simulink model "SG__MDL_IO104_IO135"  (R2022b)
settings: Solver=FixedStepAuto  StartTime=0.0  StopTime=Inf  RelTol=1e-3  EnableMultiTasking=on
model workspace (MAT data in the model file):
  a = 0.28
  ff = 1200
  fi = 150
  tmax = 40
undefined symbols (not defined in the file or in its folder): Ended, Single
libraries: dspsigops x11, simulink x8, speedgoatlib_IO135 x3, speedgoatlib_IO104 x3, hdlsllib x2, slrealtimeloglib x1, dspsrcs4 x1
settings Model: SimulationMode=external  Creator=padlewsk  LastModifiedBy=padlewsk
settings SolverCC: ConcurrentTasks=on  AlgebraicLoopSolver=TrustRegion  PositivePriorityOrder=on  AutoInsertRateTranBlk=on
settings DataIOCC: SaveFormat=StructureWithTime
settings OptimizationCC: BlockReduction=off  OptimizeBlockIOStorage=off
settings DebuggingCC: TasksWithSamePriorityMsg=none  UnconnectedInputMsg=warning  UnconnectedOutputMsg=warning  UnconnectedLineMsg=warning
settings HardwareCC: ProdBitPerLong=64  ProdLongLongMode=on  ProdHWDeviceType=Intel->x86-64 (Linux 64)
settings ModelReferenceCC: EnableRefExpFcnMdlSchedulingChecks=on
settings RTWCC: Description=Simulink Real-Time  SystemTargetFile=slrealtime.tlc  TemplateMakefile=slrealtime_default_tmf  Toolchain=Simulink Real-Time Toolchain  BuildConfiguration=Faster Runs  CodeExecutionProfiling=on  TargetLang=C++

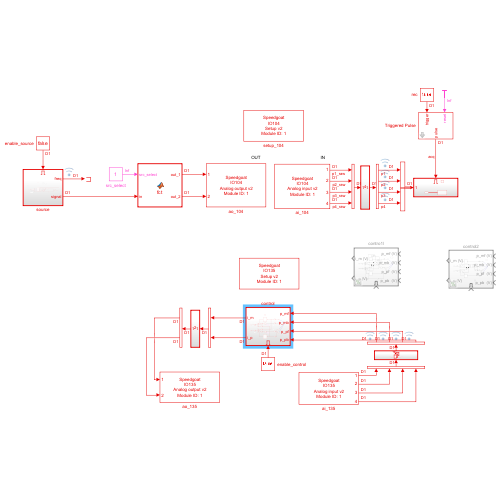
[thumbnail: Simulink's stored preview of the top-level diagram]
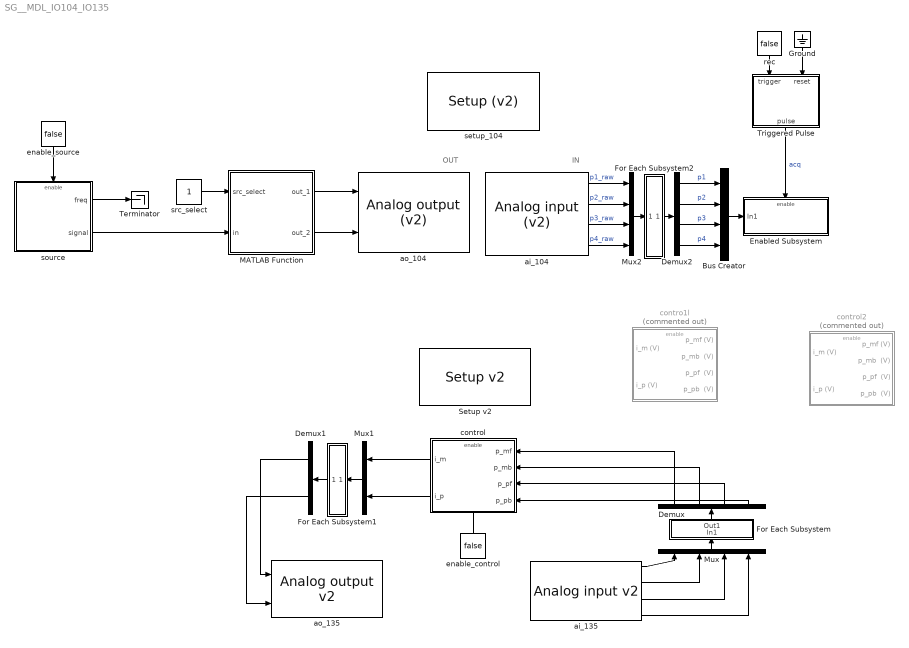
== system SG__MDL_IO104_IO135 ==
  note: IN
  note: OUT
  Bus Creator : BusCreator  Inputs=4
  Demux : Demux
  Demux1 : Demux  Outputs=2
  Demux2 : Demux
  Enabled Subsystem : Subsystem  TreatAsAtomicUnit=on
  For Each Subsystem : Subsystem  TreatAsAtomicUnit=on
  For Each Subsystem1 : Subsystem  TreatAsAtomicUnit=on
  For Each Subsystem2 : Subsystem  TreatAsAtomicUnit=on
  Ground : Ground
  MATLAB Function : MATLAB Function  TreatAsAtomicUnit=on
  Mux : Mux
  Mux1 : Mux  Inputs=2
  Mux2 : Mux
  "Setup v2 " : speedgoatlib_IO135/Setup v2   parPciSlot=-1  parModuleId=1  parInterModuleSync=None  parConvClockBaseRate=20MHz  parConvClock1Divider=20000  parConvClock2Divider=20000  parFrameTriggerEnable=off  parFrameTriggerDivider=10  parConvClock1BaseRate=1  parConvClock2BaseRate=1  parFrameTriggerClock=1  parAdcChannels=[1:4]  parAdcRange1=+-5V  parAdcRange2=+-5V  parAdcRange3=+-5V  parAdcRange4=+-5V  parAdcVoltageRange=[1 1 1 1]  parAdcOversampling1=None  parAdcOversampling2=None  parAdcOversampling3=None  parAdcOversampling4=None  parAdcOversamplRate=[1 1 1 1]  parAdcAutoCorrection=on  parAdcContSampling=off  parAdcDmaEnable=off  parAdcDmaClock=Clock 1  parAdcFrameSize_=100  parAdcSampleTime_=-1  parAdcActiveDmaDevices=[1 1 1 1]  parAdcFrameTriggerEnable=0  parAdcFrameSize=100  parAdcSampleTime=0.1  parDacChannels=[1 2]  parDacInitValues=0  parDacReset=1  parDacRange1=+-10V  parDacRange2=+-10V  parDacRange3=+-10V  parDacRange4=+-10V  parDacRange5=+-10V  parDacRange6=+-10V  parDacRange7=+-10V  parDacRange8=+-10V  parDacRange9=+-10V  parDacRange10=+-10V  parDacRange11=+-10V  parDacRange12=+-10V  parDacRange13=+-10V  parDacRange14=+-10V  parDacRange15=+-10V  parDacRange16=+-10V  parDacVoltageRange=[5 5 5 5 5 5 5 5 5 5 5 5 5 5 5 5]  parDacAutoCorrection=on  parDacSyncOut=on  parDacDmaEnable=off  parDacDmaLatency=Until next frame  parDacDmaClock=Clock 1  parDacFrameSize_=100  parDacSampleTime_=-1  parDacActiveDmaDevices=[1 1 1 1]  parDacFrameTriggerEnable=0  parDacFrameSize=100  parDacSampleTime=0.1  parDoChannels=[]  parDoInitValues=0  parDoReset=1  parDiChannels=[]  parDiDebounceEnable=off  parDiDebounceTime=0  parDiDebounceValue=0  parDioPullRefFront=Pull-up 3.3V  parDioPullRefRear=Floating
      settings: SourceProductName=Simulink Real-Time: Speedgoat I/O Blockset
  Terminator : Terminator
  Triggered Pulse : Subsystem  mask(Triggered Pulse){N=4}
      mask prompts: N "Length (N samples)"
      mask help: Generates a single pulse of N samples length
  ai_104 : speedgoatlib_IO104/Analog input (v2)   parModuleId=1  parTs=5e-05  parPciSlot=-1  parAdChannels=[1,2,3,4]  parAdChannelsSorted=[1,2,3,4]  parAdRange1=+-2.5V  parAdRange2=+-2.5V  parAdCoupling=Single-Ended  parAdFrameSize=1  parAdUseTrigger=off  parAdClockInitiator=Initiator  parAdSampleTime=9.920634921e-07  parTriggerInitiator=Initiator  parTriggerRate=4.161015625e-01
      settings: SourceProductName=Simulink Real-Time: Speedgoat I/O Blockset
  ai_135 : speedgoatlib_IO135/Analog input v2   parModuleId=1  parSampleTime=5e-05  parPciSlot=-1  parAdcChannels=[1 2 3 4]  parAdcVoltageRange=[1 1 1 1]  parAdcOversamplRate=[1 1 1 1]  parAdcContSampling=0  parAdcDmaEnable=0  parAdcActiveDmaDevices=[1 1 1 1]  parAdcFrameSize=100
      settings: SourceProductName=Simulink Real-Time: Speedgoat I/O Blockset
  ao_104 : speedgoatlib_IO104/Analog output (v2)   parModuleId=1  parTs=5e-05  parPciSlot=-1  parDaChannels=[1,2]  parDaChannelsSorted=[1,2]  parDaInitValue=[0,0]  parDaReset=[1,1]  parDaRange=+-10V  parDaFrameSize=1  parDaUseTrigger=off  parDaClockInitiator=Initiator  parDaSampleTime=9.920634921e-07  parTriggerInitiator=Initiator  parTriggerRate=4.161015625e-01  parAdBlockPresent=1
      settings: SourceProductName=Simulink Real-Time: Speedgoat I/O Blockset
  ao_135 : speedgoatlib_IO135/Analog output v2   parModuleId=1  parSampleTime=5e-05  parPciSlot=-1  parDacChannels=[1 2]  parDacVoltageRange=[5 5 5 5 5 5 5 5 5 5 5 5 5 5 5 5]  parDacInitValues=[0 0]  parDacReset=[1 1]  parDacSyncOut=1  parDacDmaEnable=0  parDacActiveDmaDevices=[1 1 1 1]  parDacDmaLatency=2  parDacFrameSize=100
      settings: SourceProductName=Simulink Real-Time: Speedgoat I/O Blockset
  contro1l : Subsystem  Commented=on
  control : Subsystem
  control2 : Subsystem  Commented=on
  enable_control : Constant  Value=false  SampleTime=-1
  enable_source : Constant  Value=false  SampleTime=-1
  rec : Constant  Value=false  SampleTime=-1
  setup_104 : speedgoatlib_IO104/Setup (v2)   parPciSlot=-1  parModuleId=1  parTriggerInitiator=Initiator  parTriggerRate=4.161015625e-01  parCalibrate=off  parAdChannels=[1:4]  parAdRange1=+-2.5V  parAdRange2=+-2.5V  parAdCoupling=Single-Ended  parAdUseTrigger=off  parAdFrameSize=1  parAdClockInitiator=Initiator  parAdSampleTime=9.920634921e-07  parDaChannels=[1:2]  parDaChannelsSorted=[1,2]  parDaInitValue=[0]  parDaReset=[1]  parDaRange=+-10V  parDaUseTrigger=off  parDaFrameSize=1  parDaClockInitiator=Initiator  parDaSampleTime=9.920634921e-07  parDioByte0Dir=Outputs  parDioByte1Dir=Inputs  parDoChannels=[]  parDoInitValues=[0]  parDoReset=[1]  parDiChannels=[]
      settings: SourceProductName=Simulink Real-Time: Speedgoat I/O Blockset
  source : Subsystem  TreatAsAtomicUnit=on
  src_select : Constant
  wires:
  enable_source/1 -> source/Enable
  Triggered Pulse/1(pulse) -> Enabled Subsystem/Enable  "acq"
  Ground/1 -> Triggered Pulse/2(reset)
  rec/1 -> Triggered Pulse/1(trigger)
  Bus Creator/1 -> Enabled Subsystem/1(In1)
  source/1(freq) -> Terminator/1
  ai_135/2 -> Mux/2
  ai_135/3 -> Mux/3
  Demux1/2 -> ao_135/2
  source/2(signal) -> MATLAB Function/2(in)
  src_select/1 -> MATLAB Function/1(src_select)
  MATLAB Function/1(out_1) -> ao_104/1
  MATLAB Function/2(out_2) -> ao_104/2
  ai_135/1 -> Mux/1
  Demux1/1 -> ao_135/1
  ai_135/4 -> Mux/4
  Mux/1 -> For Each Subsystem/1(In1)
  For Each Subsystem/1(Out1) -> Demux/1
  Mux1/1 -> For Each Subsystem1/1(In1)
  For Each Subsystem1/1(Out1) -> Demux1/1
  For Each Subsystem2/1(Out1) -> Demux2/1
  Mux2/1 -> For Each Subsystem2/1(In1)
  ai_104/1 -> Mux2/1  "p1_raw"
  ai_104/2 -> Mux2/2  "p2_raw"
  ai_104/3 -> Mux2/3  "p3_raw"
  ai_104/4 -> Mux2/4  "p4_raw"
  Demux2/2 -> Bus Creator/2  "p2"
  Demux2/1 -> Bus Creator/1  "p1"
  Demux2/3 -> Bus Creator/3  "p3"
  Demux2/4 -> Bus Creator/4  "p4"
  enable_control/1 -> control/Enable
  Demux/1 -> control/1(p_mf)
  Demux/2 -> control/2(p_mb)
  Demux/3 -> control/3(p_pf)
  Demux/4 -> control/4(p_pb)
  control/1(i_m) -> Mux1/1
  control/2(i_p) -> Mux1/2

== system SG__MDL_IO104_IO135/Enabled Subsystem ==
  In1 : Inport
  Enable : EnablePort
  File Log : slrealtimeloglib/File Log  decimation=1  inputProcessing=Elements as channels (sample based)
  wires:
  In1/1 -> File Log/1  "data"

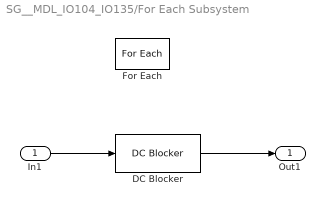
== system SG__MDL_IO104_IO135/For Each Subsystem ==
  In1 : Inport  Partition=on  PartitionDimension=1  PartitionWidth=1  PartitionOffset=0
  DC Blocker : dspsigops/DC Blocker  Algorithm=FIR  NormalizedBandwidth=0.001  Length=50  Order=6  SimulateUsing=Code generation
      settings: LibrarySourceBlock=dsphdlsupportsigops/DC Blocker
  For Each : ForEach  DisableCoverage=on
  Out1 : Outport  ConcatenationDimension=1
  wires:
  In1/1 -> DC Blocker/1
  DC Blocker/1 -> Out1/1

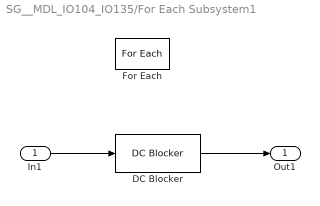
== system SG__MDL_IO104_IO135/For Each Subsystem1 ==
  In1 : Inport  Partition=on  PartitionDimension=1  PartitionWidth=1  PartitionOffset=0
  DC Blocker : dspsigops/DC Blocker  Algorithm=FIR  NormalizedBandwidth=0.001  Length=50  Order=6  SimulateUsing=Code generation
      settings: LibrarySourceBlock=dsphdlsupportsigops/DC Blocker
  For Each : ForEach  DisableCoverage=on
  Out1 : Outport  ConcatenationDimension=1
  wires:
  In1/1 -> DC Blocker/1
  DC Blocker/1 -> Out1/1

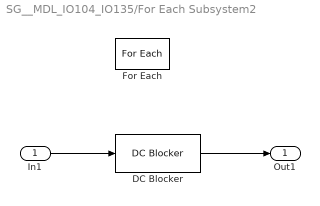
== system SG__MDL_IO104_IO135/For Each Subsystem2 ==
  In1 : Inport  Partition=on  PartitionDimension=1  PartitionWidth=1  PartitionOffset=0
  DC Blocker : dspsigops/DC Blocker  Algorithm=FIR  NormalizedBandwidth=0.001  Length=50  Order=6  SimulateUsing=Code generation
      settings: LibrarySourceBlock=dsphdlsupportsigops/DC Blocker
  For Each : ForEach  DisableCoverage=on
  Out1 : Outport  ConcatenationDimension=1
  wires:
  In1/1 -> DC Blocker/1
  DC Blocker/1 -> Out1/1

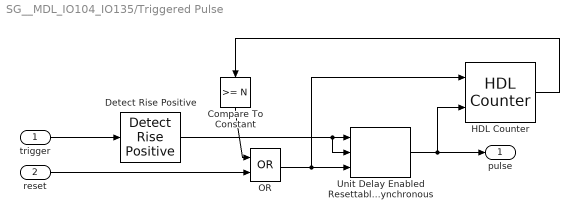
== system SG__MDL_IO104_IO135/Triggered Pulse ==
  trigger : Inport
  reset : Inport  Port=2
  Compare To Constant : simulink/Logic and Bit Operations/Compare To Constant  relop=>=  const=N  OutDataTypeStr=boolean
  Detect Rise Positive : simulink/Logic and Bit Operations/Detect Rise Positive  vinit=0  OutDataTypeStr=boolean
  HDL Counter : hdlsllib/Sources/HDL Counter  CountType=Free running  CountInit=1  CountStep=1  CountMax=25  CountFromType=Initial value  CountFrom=1  CountResetPort=on  CountLoadPort=off  CountEnbPort=on  CountDirPort=off  CountHitOutputPort=off  CountDataType=Unsigned  CountWordLen=32  CountFracLen=0  CountSampTime=1
  OR : Logic  Operator=OR  AllPortsSameDT=off  OutDataTypeStr=boolean
  Unit Delay Enabled Resettable Synchronous : hdlsllib/Discrete/Unit Delay Enabled Resettable Synchronous  InitialCondition=0.0  SampleTime=-1
  pulse : Outport  VectorParamsAs1DForOutWhenUnconnected=off
  wires:
  OR/1 -> Unit Delay Enabled Resettable Synchronous/3, HDL Counter/1
  trigger/1 -> Detect Rise Positive/1
  Unit Delay Enabled Resettable Synchronous/1 -> HDL Counter/2, pulse/1
  Compare To Constant/1 -> OR/1
  reset/1 -> OR/2
  Detect Rise Positive/1 -> Unit Delay Enabled Resettable Synchronous/1, Unit Delay Enabled Resettable Synchronous/2
  HDL Counter/1 -> Compare To Constant/1

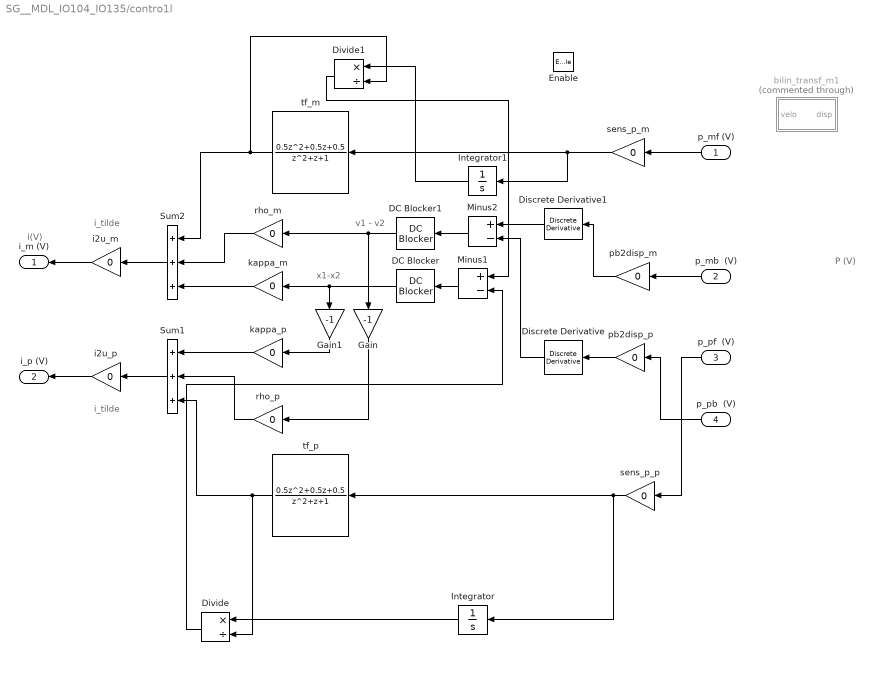
== system SG__MDL_IO104_IO135/contro1l ==
  note: v1 - v2
  note: P (V)
  note: i_tilde
  note: i(V)
  note: i_tilde
  note: x1-x2
  p_mf (V) : Inport
  p_mb  (V) : Inport  Port=2
  p_pf  (V) : Inport  Port=3
  p_pb  (V) : Inport  Port=4
  Enable : EnablePort
  DC Blocker : dspsigops/DC Blocker  Algorithm=FIR  NormalizedBandwidth=0.001  Length=50  Order=6  SimulateUsing=Code generation
      settings: LibrarySourceBlock=dsphdlsupportsigops/DC Blocker
  DC Blocker1 : dspsigops/DC Blocker  Algorithm=FIR  NormalizedBandwidth=0.001  Length=50  Order=6  SimulateUsing=Code generation
      settings: LibrarySourceBlock=dsphdlsupportsigops/DC Blocker
  Discrete Derivative : simulink/Discrete/Discrete Derivative  gainval=1.0  ICPrevScaledInput=0.0  OutMin=[]  OutMax=[]  OutDataType=fixdt(1, 16)  OutScaling=2^-10  DoSatur=off
  Discrete Derivative1 : simulink/Discrete/Discrete Derivative  gainval=1.0  ICPrevScaledInput=0.0  OutMin=[]  OutMax=[]  OutDataType=fixdt(1, 16)  OutScaling=2^-10  DoSatur=off
  Divide : Product  Inputs=*/
  Divide1 : Product  Inputs=*/
  Gain : Gain  Gain=-1
  Gain1 : Gain  Gain=-1
  Integrator : Integrator
  Integrator1 : Integrator
  Minus1 : Sum  Inputs=+-
  Minus2 : Sum  Inputs=+-
  Sum1 : Sum  Inputs=+++
  Sum2 : Sum  Inputs=+++
  bilin_transf_m1 : Subsystem  Commented=through
  i2u_m : Gain  Gain=0
  i2u_p : Gain  Gain=0
  kappa_m : Gain  Gain=0
  kappa_p : Gain  Gain=0
  pb2disp_m : Gain  Gain=0
  pb2disp_p : Gain  Gain=0
  rho_m : Gain  Gain=0
  rho_p : Gain  Gain=0
  sens_p_m : Gain  Gain=0
  sens_p_p : Gain  Gain=0
  tf_m : DiscreteTransferFcn  Numerator="[0.5         0.5         0.5]"  Denominator="[1  1  1]"
  tf_p : DiscreteTransferFcn  Numerator="[0.5         0.5         0.5]"  Denominator="[1  1  1]"
  i_m (V) : Outport
  i_p (V) : Outport  Port=2
  wires:
  p_mb  (V)/1 -> pb2disp_m/1
  p_pf  (V)/1 -> sens_p_p/1
  p_pb  (V)/1 -> pb2disp_p/1
  p_mf (V)/1 -> sens_p_m/1
  sens_p_m/1 -> Integrator1/1, tf_m/1
  sens_p_p/1 -> Integrator/1, tf_p/1
  i2u_m/1 -> i_m (V)/1
  i2u_p/1 -> i_p (V)/1
  pb2disp_p/1 -> Discrete Derivative/1
  pb2disp_m/1 -> Discrete Derivative1/1
  Minus2/1 -> DC Blocker1/1
  Discrete Derivative/1 -> Minus2/2
  Gain/1 -> rho_p/1
  Gain1/1 -> kappa_p/1
  rho_p/1 -> Sum1/2
  tf_p/1 -> Divide/2, Sum1/3
  kappa_p/1 -> Sum1/1
  Sum1/1 -> i2u_p/1
  kappa_m/1 -> Sum2/3
  rho_m/1 -> Sum2/2
  Discrete Derivative1/1 -> Minus2/1
  tf_m/1 -> Divide1/2, Sum2/1
  Sum2/1 -> i2u_m/1
  DC Blocker/1 -> Gain1/1, kappa_m/1
  DC Blocker1/1 -> rho_m/1, Gain/1
  Integrator/1 -> Divide/1
  Divide/1 -> Minus1/2
  Integrator1/1 -> Divide1/1
  Minus1/1 -> DC Blocker/1
  Divide1/1 -> Minus1/1

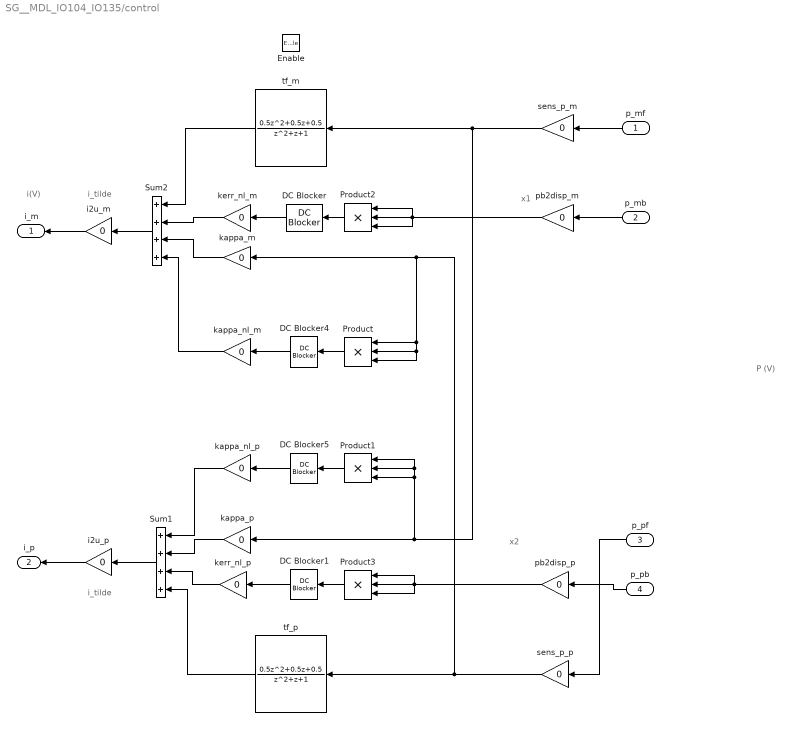
== system SG__MDL_IO104_IO135/control ==
  note: x2
  note: P (V)
  note: i_tilde
  note: i(V)
  note: i_tilde
  note: x1
  p_mf : Inport
  p_mb : Inport  Port=2
  p_pf : Inport  Port=3
  p_pb : Inport  Port=4
  Enable : EnablePort
  DC Blocker{,1,4..5} (4 alike) : dspsigops/DC Blocker  Algorithm=FIR  NormalizedBandwidth=0.001  Length=50  Order=6  SimulateUsing=Code generation
      settings: LibrarySourceBlock=dsphdlsupportsigops/DC Blocker
  Product{,1..3} (4 alike) : Product  Inputs=3
  Sum1 : Sum  Inputs=++++
  Sum2 : Sum  Inputs=++++
  i2u_m : Gain  Gain=0
  i2u_p : Gain  Gain=0
  kappa_m : Gain  Gain=0
  kappa_nl_m : Gain  Gain=0
  kappa_nl_p : Gain  Gain=0
  kappa_p : Gain  Gain=0
  kerr_nl_m : Gain  Gain=0
  kerr_nl_p : Gain  Gain=0
  pb2disp_m : Gain  Gain=0
  pb2disp_p : Gain  Gain=0
  sens_p_m : Gain  Gain=0
  sens_p_p : Gain  Gain=0
  tf_m : DiscreteTransferFcn  Numerator="[0.5         0.5         0.5]"  Denominator="[1  1  1]"
  tf_p : DiscreteTransferFcn  Numerator="[0.5         0.5         0.5]"  Denominator="[1  1  1]"
  i_m : Outport
  i_p : Outport  Port=2
  wires:
  p_pf/1 -> sens_p_p/1
  p_pb/1 -> pb2disp_p/1
  p_mf/1 -> sens_p_m/1
  i2u_m/1 -> i_m/1
  i2u_p/1 -> i_p/1
  kerr_nl_p/1 -> Sum1/3
  tf_p/1 -> Sum1/4
  Sum1/1 -> i2u_p/1
  kerr_nl_m/1 -> Sum2/2
  tf_m/1 -> Sum2/1
  Sum2/1 -> i2u_m/1
  Product3/1 -> DC Blocker1/1
  Product2/1 -> DC Blocker/1
  DC Blocker/1 -> kerr_nl_m/1
  DC Blocker1/1 -> kerr_nl_p/1
  p_mb/1 -> pb2disp_m/1
  sens_p_m/1 -> tf_m/1, kappa_p/1, Product1/1, Product1/2, Product1/3
  sens_p_p/1 -> Product/3, Product/2, Product/1, kappa_m/1, tf_p/1
  kappa_m/1 -> Sum2/3
  kappa_p/1 -> Sum1/2
  Product1/1 -> DC Blocker5/1
  DC Blocker4/1 -> kappa_nl_m/1
  kappa_nl_m/1 -> Sum2/4
  DC Blocker5/1 -> kappa_nl_p/1
  kappa_nl_p/1 -> Sum1/1
  Product/1 -> DC Blocker4/1
  pb2disp_p/1 -> Product3/3, Product3/1, Product3/2
  pb2disp_m/1 -> Product2/1, Product2/3, Product2/2

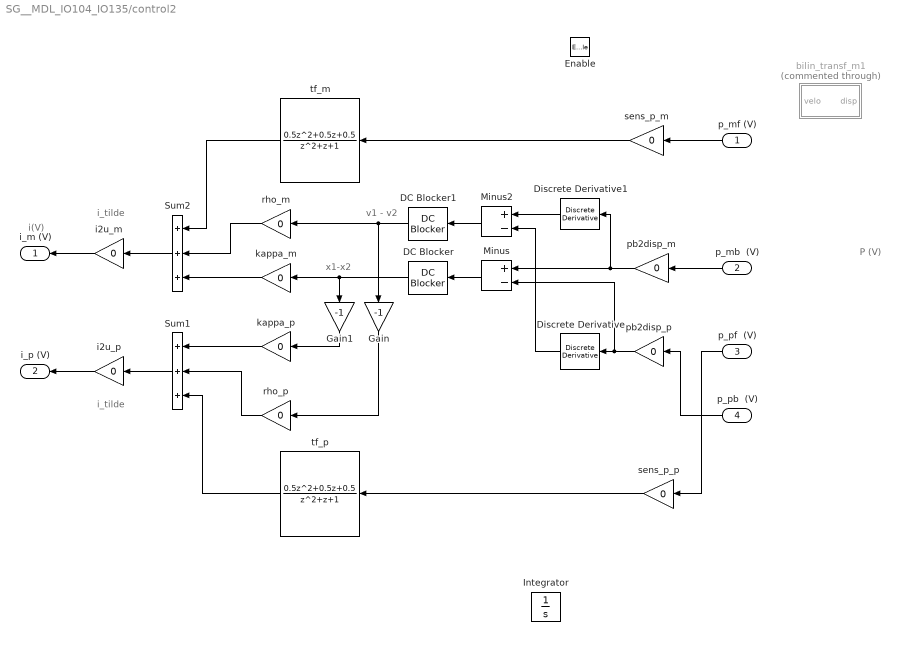
== system SG__MDL_IO104_IO135/control2 ==
  note: v1 - v2
  note: P (V)
  note: i_tilde
  note: i(V)
  note: i_tilde
  note: x1-x2
  p_mf (V) : Inport
  p_mb  (V) : Inport  Port=2
  p_pf  (V) : Inport  Port=3
  p_pb  (V) : Inport  Port=4
  Enable : EnablePort
  DC Blocker : dspsigops/DC Blocker  Algorithm=FIR  NormalizedBandwidth=0.001  Length=50  Order=6  SimulateUsing=Code generation
      settings: LibrarySourceBlock=dsphdlsupportsigops/DC Blocker
  DC Blocker1 : dspsigops/DC Blocker  Algorithm=FIR  NormalizedBandwidth=0.001  Length=50  Order=6  SimulateUsing=Code generation
      settings: LibrarySourceBlock=dsphdlsupportsigops/DC Blocker
  Discrete Derivative : simulink/Discrete/Discrete Derivative  gainval=1.0  ICPrevScaledInput=0.0  OutMin=[]  OutMax=[]  OutDataType=fixdt(1, 16)  OutScaling=2^-10  DoSatur=off
  Discrete Derivative1 : simulink/Discrete/Discrete Derivative  gainval=1.0  ICPrevScaledInput=0.0  OutMin=[]  OutMax=[]  OutDataType=fixdt(1, 16)  OutScaling=2^-10  DoSatur=off
  Gain : Gain  Gain=-1
  Gain1 : Gain  Gain=-1
  Integrator : Integrator
  Minus : Sum  Inputs=+-
  Minus2 : Sum  Inputs=+-
  Sum1 : Sum  Inputs=+++
  Sum2 : Sum  Inputs=+++
  bilin_transf_m1 : Subsystem  Commented=through
  i2u_m : Gain  Gain=0
  i2u_p : Gain  Gain=0
  kappa_m : Gain  Gain=0
  kappa_p : Gain  Gain=0
  pb2disp_m : Gain  Gain=0
  pb2disp_p : Gain  Gain=0
  rho_m : Gain  Gain=0
  rho_p : Gain  Gain=0
  sens_p_m : Gain  Gain=0
  sens_p_p : Gain  Gain=0
  tf_m : DiscreteTransferFcn  Numerator="[0.5         0.5         0.5]"  Denominator="[1  1  1]"
  tf_p : DiscreteTransferFcn  Numerator="[0.5         0.5         0.5]"  Denominator="[1  1  1]"
  i_m (V) : Outport
  i_p (V) : Outport  Port=2
  wires:
  p_mb  (V)/1 -> pb2disp_m/1
  p_pf  (V)/1 -> sens_p_p/1
  p_pb  (V)/1 -> pb2disp_p/1
  p_mf (V)/1 -> sens_p_m/1
  sens_p_m/1 -> tf_m/1
  sens_p_p/1 -> tf_p/1
  i2u_m/1 -> i_m (V)/1
  i2u_p/1 -> i_p (V)/1
  pb2disp_p/1 -> Minus/2, Discrete Derivative/1
  pb2disp_m/1 -> Minus/1, Discrete Derivative1/1
  Minus2/1 -> DC Blocker1/1
  Discrete Derivative/1 -> Minus2/2
  Minus/1 -> DC Blocker/1
  Gain/1 -> rho_p/1
  Gain1/1 -> kappa_p/1
  rho_p/1 -> Sum1/2
  tf_p/1 -> Sum1/3
  kappa_p/1 -> Sum1/1
  Sum1/1 -> i2u_p/1
  kappa_m/1 -> Sum2/3
  rho_m/1 -> Sum2/2
  Discrete Derivative1/1 -> Minus2/1
  tf_m/1 -> Sum2/1
  Sum2/1 -> i2u_m/1
  DC Blocker/1 -> Gain1/1, kappa_m/1
  DC Blocker1/1 -> rho_m/1, Gain/1

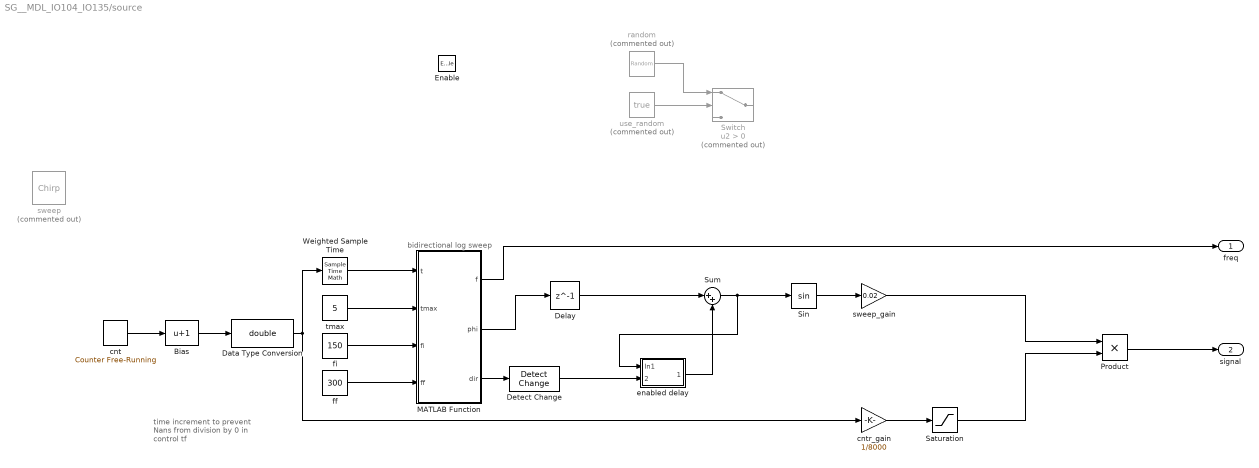
== system SG__MDL_IO104_IO135/source ==
  note: bidirectional log sweep
  note: time increment to prevent Nans from division by 0 in control tf
  Enable : EnablePort  StatesWhenEnabling=reset
  Bias : Bias  Bias=1  SaturateOnIntegerOverflow=off
  Data Type Conversion : DataTypeConversion  OutDataTypeStr=double  SaturateOnIntegerOverflow=off  RndMeth=Floor
  Delay : Delay  DelayLength=1
  Detect Change : simulink/Logic and Bit Operations/Detect Change  vinit=false  OutDataTypeStr=boolean
  MATLAB Function : MATLAB Function  TreatAsAtomicUnit=on
  Product : Product
  Saturation : Saturate  UpperLimit=1  LowerLimit=0
  Sin : Trigonometry
  Sum : Sum  Inputs=|++
  Switch : Switch  Commented=on  Criteria=u2 > Threshold  SaturateOnIntegerOverflow=off  InputSameDT=off
  Weighted Sample Time : SampleTimeMath  TsampMathOp=*
  cnt : simulink/Sources/Counter Free-Running  NumBits=32  tsamp=-1
  cntr_gain : Gain  Gain=1/8000  ParamDataTypeStr=double
  enabled delay : Subsystem
  ff : Constant  Value=300
  fi : Constant  Value=150
  random : RandomNumber  Commented=on  Variance=0.5  SampleTime=3.5e-05
  sweep : dspsrcs4/Chirp  Commented=on  sweep=Logarithmic  mode=Bidirectional  f0=150  f1=1200  t1=10  Tsweep=20  phase=0  Ts=3.5e-05  spf=1  datatype=Double  OutputFrames=off
  sweep_gain : Gain  Gain=0.02
  tmax : Constant  Value=5
  use_random : Constant  Commented=on  Value=true  SampleTime=-1
  freq : Outport  OutputWhenDisabled=reset  InitialOutput=0  VectorParamsAs1DForOutWhenUnconnected=off
  signal : Outport  Port=2  OutputWhenDisabled=reset  InitialOutput=0  VectorParamsAs1DForOutWhenUnconnected=off
  wires:
  use_random/1 -> Switch/2
  random/1 -> Switch/1
  sweep_gain/1 -> Product/1
  cntr_gain/1 -> Saturation/1
  Product/1 -> signal/1
  MATLAB Function/2(phi) -> Delay/1
  Saturation/1 -> Product/2
  Weighted Sample Time/1 -> MATLAB Function/1(t)
  Data Type Conversion/1 -> cntr_gain/1, Weighted Sample Time/1
  MATLAB Function/1(f) -> freq/1
  Sin/1 -> sweep_gain/1
  MATLAB Function/3(dir) -> Detect Change/1
  Detect Change/1 -> enabled delay/2(enable)
  Delay/1 -> Sum/1
  enabled delay/1(Out1) -> Sum/2
  Sum/1 -> enabled delay/1(In1), Sin/1
  cnt/1 -> Bias/1
  Bias/1 -> Data Type Conversion/1
  ff/1 -> MATLAB Function/4(ff)
  tmax/1 -> MATLAB Function/2(tmax)
  fi/1 -> MATLAB Function/3(fi)

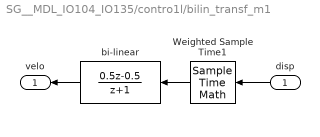
== system SG__MDL_IO104_IO135/contro1l/bilin_transf_m1 ==
  disp : Inport
  Weighted Sample Time1 : SampleTimeMath  TsampMathOp=/
  "bi-linear " : DiscreteTransferFcn  Numerator=[0.5, -0.5]  Denominator=[1, 1]
  velo : Outport
  wires:
  disp/1 -> Weighted Sample Time1/1
  Weighted Sample Time1/1 -> "bi-linear "/1
  "bi-linear "/1 -> velo/1

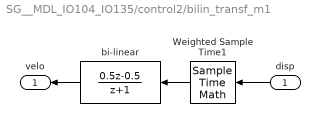
== system SG__MDL_IO104_IO135/control2/bilin_transf_m1 ==
  disp : Inport
  Weighted Sample Time1 : SampleTimeMath  TsampMathOp=/
  "bi-linear " : DiscreteTransferFcn  Numerator=[0.5, -0.5]  Denominator=[1, 1]
  velo : Outport
  wires:
  disp/1 -> Weighted Sample Time1/1
  Weighted Sample Time1/1 -> "bi-linear "/1
  "bi-linear "/1 -> velo/1

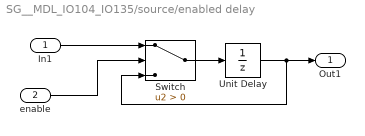
== system SG__MDL_IO104_IO135/source/enabled delay ==
  In1 : Inport
  enable : Inport  Port=2
  Switch : Switch  Criteria=u2 > Threshold  SaturateOnIntegerOverflow=off  InputSameDT=off
  Unit Delay : UnitDelay  SampleTime=-1  HasFrameUpgradeWarning=on
  Out1 : Outport
  wires:
  Unit Delay/1 -> Switch/3, Out1/1
  Switch/1 -> Unit Delay/1
  In1/1 -> Switch/1
  enable/1 -> Switch/2

== matlab function SG__MDL_IO104_IO135/MATLAB Function ==
  data: src_select input; in input; out_1 output; out_2 output
function [out_1, out_2] = fct(src_select, in)
out_1 = 0;
out_2 = 0;
if src_select == 1
    out_1 = in;
elseif src_select == 2
    out_2 = in;
end

== matlab function SG__MDL_IO104_IO135/source/MATLAB Function ==
  data: f output; t input; tmax input; phi output; dir output; fi input; ff input
function [f, phi, dir] = fcn(t, tmax, fi, ff)
%tmax is the time at which the maximum frequency is reached

t = mod(t, 2*tmax);

if t < tmax
    % up
    dir = 1;
    
    
    % linear (CF wikipedia)
%     phi = 2*pi*(0.5*(ff - fi)*t^2/tmax + fi*t);
%     f = fi + (ff - fi)*t/tmax;
    
    % logarithmic %%% https://en.wikipedia.org/wiki/Chirp
    k = log((ff/fi)^(1/tmax));
    phi = 2*pi*fi*(exp(k*t) - 1)/k;
    f = fi*exp(k*t);
else
    % down
    dir = -1;
    
    
    % linear (CF wikipedia)
%     phi = 2*pi*(0.5*(fi - ff)*(t-tmax)^2/tmax + ff*(t-tmax)); % linear
%     f = ff + (fi - ff)*(t - tmax)/tmax;
    
    % logarithmic
    k = log((fi/ff)^(1/tmax));
    phi = 2*pi*ff*(exp(k*(t - tmax)) - 1)/k;
    f = ff*exp(k*(t-tmax));
end

phi = mod(phi, 2*pi);
